simulink library "commdigpbnd"  (Simulink 5.0)
undefined symbols (not defined in the file or in its folder): j, Offset, T
libraries: commdigbbnd x13, commanapbnd x11, commutil x9, commdigpbnd x3, commsource x1
settings Model: Creator=tdelve  LastModifiedBy=mmclerno

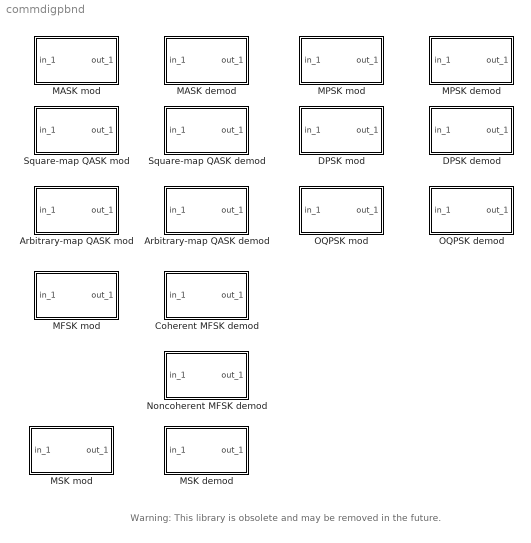
== system commdigpbnd ==
  note: Warning: This library is obsolete and may be removed in the future.
  Arbitrary-map QASK demod : Subsystem  mask(Passband A-map QASK demodulation){y1=real(exp(j*[0:8-1]/8*pi*2)), y2=imag(exp(j*[0:8-1]/8*pi*2)), td=0.1, Fc=100, Ph=0, ts=0.001}
      mask prompts: y1 "Vector of in-phase component:"; y2 "Vector of quadrature component:"; td "Symbol interval (sec):"; Fc "Carrier frequency (Hz):"; Ph "Initial phase (rad):"; ts "Sample time (sec):"
      mask help: Demodulate a QASK modulated signal with user-defined arbitrary constellation.
      mask init:
      | [num,den]=butter(5,Fc*2*ts);
      mask Help: This block demodulates a QASK modulated signal using user-defined arbitrary constellation. The arbitrary defined map is given in in-phase and quadrature component vector. The vector length of in-phase and quadrature components should have the same length. This block uses a default lowpass filter, which is [num,den]=butter(5,Fc*2*ts). Ungroup this block to define your own filter.
      mask Display:
      | plot(0,0,100,100,[5+1.5*[[0:.8:10] [10 20] [20:.8:30]] 50 50 50 50+15*[0 1 1 2 2 3]],[85+10*[sin([0:.8:10]*pi*2/5) 0 0 sin([20:.8:30]*pi*2/5)] 85 99 75 85+8*[1 1 -1 -1 1 1]]);
      | disp('\nPassband\nA-QASK')
  Arbitrary-map QASK mod : Subsystem  mask(Passband A-map QASK modulation){y1=real(exp(j*[0:8-1]/8*pi*2)), y2=imag(exp(j*[0:8-1]/8*pi*2)), td=0.1, Fc=100, Ph=0, ts=0.001}
      mask prompts: y1 "Vector of in-phase component:"; y2 "Vector of quadrature component:"; td "Symbol interval (sec):"; Fc "Carrier frequency (Hz):"; Ph "Initial phase (rad):"; ts "Sample time (sec):"
      mask help: Modulate the input digital signal using quadrature amplitude shift keying method with arbitrary constellation.
      mask Help: This block modulates a digital signal using QASK method with user-defined arbitrary constellation. The vector length of the in-phase and quadrature components vector should have the same length. The inputs are integers in the range [0, M-1], where M is the M-ary number. When the symbol interval is a two-element vector, the second element is the offset (default 0).
      mask Display:
      | plot(0,0,100,100,[5+15*[0 1 1 2 2 3] 50 50 50 50+1.5*[[0:.8:10] [10 20] [20:.8:30]]],[85+8*[1 1 -1 -1 1 1] 85 99 75 85+10*[sin([0:.8:10]*pi*2/5) 0 0 sin([20:.8:30]*pi*2/5)]]);
      | disp('\nPassband\nA-QASK')
  Coherent MFSK demod : Subsystem  mask(Passband MFSK demodulation){M=8, Ton=8/.1/5, td=0.1, Fc=100, Ph=0, ts=0.001}
      mask prompts: M "M-ary number (output digits in range [0, M-1]):"; Ton "Tone space (Hz):"; td "Symbol interval (sec):"; Fc "Carrier frequency (Hz):"; Ph "Initial phase (rad):"; ts "Sample time (sec):"
      mask help: Demodulate a MFSK modulated signal using coherent demodulation method.
      mask Help: This block demodulates a MFSK modulated signal using coherent method. The coherence demodulation method is phase sensitive. The tone space is the frequency distance between two consecutive digit after the modulation. The inputs are integers in the range [0, M-1], where M is the M-ary number. When the symbol interval is a two-element vector, the second element is the offset (default 0).
      mask Display:
      | plot(0,0,100,100,[5+1.5*[[0:.8:10] [10:1.6:20] [20:.8:30]] 50 50 50 50+15*[0 1 1 2 2 3]],[85+10*[sin([0:.8:10]*pi*2/5) sin([10:1.6:20]*pi/5) sin([20:.8:30]*pi*2/5)] 85 99 75 85+8*[1 1 -1 -1 1 1]]);
      | disp('\nPassband\nCohe MFSK')
  DPSK demod : Subsystem  mask(Passband DPSK demodulation){td=0.1, Fc=100, Ph=0, ts=0.001}
      mask prompts: td "Symbol interval (sec):"; Fc "Carrier frequency (Hz):"; Ph "Initial phase (rad):"; ts "Sample time (sec):"
      mask help: Demodulate a DPSK modulated signal.
      mask Help: This block demodulates a DPSK modulated signal using the digital MPSK Demod block and the Differential Decoder block. The input is a modulated analog signal and the output is a demodulated binary signal. Match the parameters to the ones used in the corresponding DPSK Mod block. The offset value in Symbol interval can be different.
      mask Display:
      | plot(0,0,100,100,[5+1.5*[[0:.8:10] [10:1.6:20] [20:.8:30]] 50 50 50 50+15*[0 1 1 2 2 3]],[85+10*[sin([0:.8:10]*pi*2/5) sin([10:1.6:20]*pi/5) sin([20:.8:30]*pi*2/5)] 85 99 75 85+8*[1 1 -1 -1 1 1]]);
      | disp('\nPassband\nDPSK')
  DPSK mod : Subsystem  mask(Passband DPSK modulation){td=0.1, Fc=100, Ph=0, ts=0.001}
      mask prompts: td "Symbol interval (sec):"; Fc "Carrier frequency (Hz):"; Ph "Initial phase (rad):"; ts "Sample time (sec):"
      mask help: Modulate the input signal using differential phase shift keying method.
      mask Help: This block modulates a digital signal with a given carrier frequency using the DPSK method. The input to this block is a binary signal. When the symbol interval is a two-element vector, the second element is the offset (default is 0). The output is a modulated analog signal with a maximum amplitude equal to 1.
      mask Display:
      | plot(0,0,100,100,[5+15*[0 1 1 2 2 3] 50 50 50 50+1.5*[[0:.8:10] [10:1.6:20] [20:.8:30]]],[85+8*[1 1 -1 -1 1 1] 85 99 75 85+10*[sin([0:.8:10]*pi*2/5) sin([10:1.6:20]*pi/5) sin([20:.8:30]*pi*2/5)]]);
      | disp('\nPassband\nDPSK')
  MASK demod : Subsystem  mask(Passband MASK demodulation){M=8, td=0.1, Fc=100, Ph=0, ts=0.001}
      mask prompts: M "M-ary number (output integer in range [0, M-1]):"; td "Symbol interval (sec):"; Fc "Carrier Frequency (Hz):"; Ph "Initial phase (rad):"; ts "Sample time (sec):"
      mask help: Demodulate a MASK modulated signal.
      mask init:
      | [num,den]=butter(5,Fc*2*ts);
      mask Help: This block demodulates a MASK modulated signal. The output signals are digits in range [0, M-1]. When the symbol interval is a two element vector, the second element is the offset (default 0). A default lowpass filter is used in the demodulation, which is [num, den]=butter(5, Fc*2*ts). Ungroup this block to specify the numerator and denominator of the lowpass filter.
      mask Display:
      | plot(0,0,100,100,[5+1.5*[[0:.8:10] [10 20] [20:.8:30]] 50 50 50 50+15*[0 1 1 2 2 3]],[85+10*[sin([0:.8:10]*pi*2/5) 0 0 sin([20:.8:30]*pi*2/5)] 85 99 75 85+8*[1 1 -1 -1 1 1]]);
      | disp('\nPassband\nMASK');
  MASK mod : Subsystem  mask(Passband MASK modulation){M=8, td=0.1, Fc=100, Ph=0, ts=0.001}
      mask prompts: M "M-ary number (input integer in range [0, M-1]):"; td "Input symbol interval (sec):"; Fc "Carrier frequency (Hz):"; Ph "Carrier initial phase (rad):"; ts "Sample time (sec):"
      mask help: Modulate the input digital signal using M-ary amplitude shift keying method.
      mask Help: This block modulates a digital signal using MASK method. The inputs are integers in the range [0, M-1], where M is the M-ary number. When the symbol interval is a two-element vector, the second element is the offset (default 0). The block keeps the input value at the offset time point for the entire interval.
      mask Display:
      | plot(0,0,100,100,[5+15*[0 1 1 2 2 3] 50 50 50 50+1.5*[[0:.8:10] [10 20] [20:.8:30]]],[85+8*[1 1 -1 -1 1 1] 85 99 75 85+10*[sin([0:.8:10]*pi*2/5) 0 0 sin([20:.8:30]*pi*2/5)]]);
      | disp('\nPassband\nMASK')
  MFSK mod : Subsystem  mask(Passband FSK modulation){Ton=8/.1/5, td=0.1, Fc=100, Ph=0, ts=0.001}
      mask prompts: Ton "Tone space(Hz):"; td "Symbol interval (sec):"; Fc "Carrier frequency (Hz):"; Ph "Initial phase (rad):"; ts "Sample time (sec):"
      mask help: Modulate the input digital signal using M-ary frequency shift keying method.
      mask Help: This block modulates a digital signal using FSK method. The modulation resets the modulation phase to be the specified initial phase at the beginning of each digit. Tone space is the frequency distance between two consecutive digits after modulation. The output signal has its frequency in the range [Fc, Fc + Tone_space*Max_In_Value], where Fc is the carrier frequency.
      mask Display:
      | plot(0,0,100,100,[5+15*[0 1 1 2 2 3] 50 50 50 50+1.5*[[0:.8:10] [10:1.6:20] [20:.8:30]]],[85+8*[1 1 -1 -1 1 1] 85 99 75 85+10*[sin([0:.8:10]*pi*2/5) sin([10:1.6:20]*pi/5) sin([20:.8:30]*pi*2/5)]]);
      | disp('\nPassband\nMFSK');
  MPSK demod : Subsystem  mask(Passband MPSK demodulation){M=8, td=0.1, Fc=100, Ph=0, ts=0.001}
      mask prompts: M "M-ary number (output integer in range [0, M-1]):"; td "Symbol interval (sec):"; Fc "Carrier frequency (Hz):"; Ph "Initial phase (rad):"; ts "Sample time (sec):"
      mask help: Demodulate a MPSK modulated signal using correlation method.
      mask Help: This block demodulates a MPSK modulated signal using correlation method. The output signals are digits in range [0, M-1], where M is the M-ary number. When the symbol interval is a two-element vector, the second element is the offset (default 0).
      mask Display:
      | plot(0,0,100,100,[5+1.5*[[0:.8:10] [10:1.6:20] [20:.8:30]] 50 50 50 50+15*[0 1 1 2 2 3]],[85+10*[sin([0:.8:10]*pi*2/5) sin([10:1.6:20]*pi/5) sin([20:.8:30]*pi*2/5)] 85 99 75 85+8*[1 1 -1 -1 1 1]]);
      | disp('\nPassband\nMPSK')
  MPSK mod : Subsystem  mask(Passband MPSK modulation){M=8, td=0.1, Fc=100, Ph=0, ts=0.001}
      mask prompts: M "M-ary number (input integer in range [0, M-1]):"; td "Symbol interval (sec):"; Fc "Carrier frequency (Hz):"; Ph "Initial phase (rad):"; ts "Sample time (sec):"
      mask help: Modulate the input signal using M-ary phase shift keying method.
      mask Help: This block modulates a digital signal with a given carrier frequency using MPSK method. The inputs are integers in the range [0, M-1], where M is the M-ary number. When the symbol interval is a two element vector, the second element is the offset (default 0). The block keeps the input value at the offset time point for the entire interval.
      mask Display:
      | plot(0,0,100,100,[5+15*[0 1 1 2 2 3] 50 50 50 50+1.5*[[0:.8:10] [10:1.6:20] [20:.8:30]]],[85+8*[1 1 -1 -1 1 1] 85 99 75 85+10*[sin([0:.8:10]*pi*2/5) sin([10:1.6:20]*pi/5) sin([20:.8:30]*pi*2/5)]]);
      | disp('\nPassband\nMPSK')
  MSK demod : Subsystem  mask(Passband MSK demodulation){td=0.1, Fc=100, Ph=0, ts=0.001}
      mask prompts: td "Symbol interval (sec):"; Fc "Carrier frequency (Hz):"; Ph "Initial phase (rad):"; ts "Sample time (sec):"
      mask help: Demodulate an MSK modulated signal.
      mask init:
      | T(1)=td(1);T2=2*T(1);if length(td)>1,T(2)=td(2); else, T(2)=0;end
      mask Help: This block demodulates an MSK modulated signal. It uses a matched filter to process the input signal and detect the in-phase and quadrature components of the signal. The filtered output is fed to an OQPSK Demap block resulting in a binary signal. Match the parameters to the ones used in the corresponding MSK Mod block. The offset value in Symbol interval can be different.
      mask Display:
      | plot(0,0,100,100,[5+1.5*[[0:.8:10] [10 20] [20:.8:30]] 50 50 50 50+15*[0 1 1 2 2 3]],[85+10*[sin([0:.8:10]*pi*2/5) 0 0 sin([20:.8:30]*pi*2/5)] 85 99 75 85+8*[1 1 -1 -1 1 1]]);
      | disp('\nPassband\nMSK')
  MSK mod : Subsystem  mask(Passband MSK modulation){td=0.1, Fc=100, Ph=0, ts=0.001}
      mask prompts: td "Symbol interval (sec):"; Fc "Carrier frequency (Hz):"; Ph "Initial phase (rad):"; ts "Sample time (sec):"
      mask help: Modulate the input signal using minimum phase shift keying method.
      mask Help: This block modulates a digital signal with a given carrier frequency using the MSK method. It uses the OQPSK Map block to map the binary input signal to the in-phase and quadrature components. When the symbol interval is a two-element vector, the second element is the offset (default is 0). The output is a modulated analog signal with a maximum amplitude equal to 1.
      mask Display:
      | plot(0,0,100,100,[5+15*[0 1 1 2 2 3] 50 50 50 50+1.5*[[0:.8:10] [10:1.6:20] [20:.8:30]]],[85+8*[1 1 -1 -1 1 1] 85 99 75 85+10*[sin([0:.8:10]*pi*2/5) sin([10:1.6:20]*pi/5) sin([20:.8:30]*pi*2/5)]]);
      | disp('\nPassband\nMSK')
  Noncoherent MFSK demod : Subsystem  mask(Passband MPSK demodulation){M=8, Ton=8/.1/5, td=0.1, Fc=100, Ph=pi/6, ts=0.001}
      mask prompts: M "M-ary number (output digits in range [0, M-1]):"; Ton "Tone space (Hz):"; td "Symbol interval (sec):"; Fc "Carrier frequency (Hz):"; Ph "Initial phase (rad):"; ts "Sample time (sec):"
      mask help: Demodulate a MFSK modulated signal using noncoherent method.
      mask Help: This block demodulates a MFSK modulated signal using noncoherent method. The tone space is the frequency distance between two consecutive after the modulation. The inputs are integers in the range [0, M-1], where M is the M-ary number. When the symbol interval is a two-element vector, the second element is the offset (default 0).
      mask Display:
      | plot(0,0,100,100,[5+1.5*[[0:.8:10] [10:1.6:20] [20:.8:30]] 50 50 50 50+15*[0 1 1 2 2 3]],[85+10*[sin([0:.8:10]*pi*2/5) sin([10:1.6:20]*pi/5) sin([20:.8:30]*pi*2/5)] 85 99 75 85+8*[1 1 -1 -1 1 1]]);
      | disp('\nPassband\nNonc MFSK')
  OQPSK demod : Subsystem  mask(Passband OQPSK demodulation){td=0.1, Fc=100, Ph=0, ts=0.001}
      mask prompts: td "Symbol interval (sec):"; Fc "Carrier frequency (Hz):"; Ph "Initial phase (rad):"; ts "Sample time (sec):"
      mask help: Demodulate an OQPSK modulated signal.
      mask init:
      | [num,den]=butter(5,Fc*2*ts);NIR=4;AIR=1/sqrt(2);PIR=pi/4;
      mask Help: This block demodulates an OQPSK modulated signal. The inputs are the in-phase and quadrature components of the QAM demodulated (QADM) signal. The output is a scalar binary signal with sample time T.
      mask Display:
      | plot(0,0,100,100,[5+1.5*[[0:.8:10] [10 20] [20:.8:30]] 50 50 50 50+15*[0 1 1 2 2 3]],[85+10*[sin([0:.8:10]*pi*2/5) 0 0 sin([20:.8:30]*pi*2/5)] 85 99 75 85+8*[1 1 -1 -1 1 1]]);
      | disp('\nPassband\nOQPSK')
  OQPSK mod : Subsystem  mask(Passband OQPSK modulation){td=0.1, Fc=100, Ph=0, ts=0.001}
      mask prompts: td "Symbol interval (sec):"; Fc "Carrier frequency (Hz):"; Ph "Initial phase (rad):"; ts "Sample time (sec):"
      mask help: Modulate the input signal using offset quadrature phase shift keying method.
      mask Help: This block modulates a digital signal with a given carrier frequency using the OQPSK method. The input to this block is a binary signal. When the symbol interval is a two-element vector, the second element is the offset (default is 0). The block uses the OQPSK Map block before feeding the signal to the QAM block. The output is a modulated analog signal with maximum amplitude equal to 1.
      mask Display:
      | plot(0,0,100,100,[5+15*[0 1 1 2 2 3] 50 50 50 50+1.5*[[0:.8:10] [10:1.6:20] [20:.8:30]]],[85+8*[1 1 -1 -1 1 1] 85 99 75 85+10*[sin([0:.8:10]*pi*2/5) sin([10:1.6:20]*pi/5) sin([20:.8:30]*pi*2/5)]]);
      | disp('\nPassband\nOQPSK')
  Square-map QASK demod : Subsystem  mask(Passband S-QASK demodulation){M=8, td=0.1, Fc=100, Ph=0, ts=0.001}
      mask prompts: M "M-ary number (output integer in range [0 M-1]):"; td "Symbol interval (sec):"; Fc "Carrier Frequency (Hz):"; Ph "Initial phase (rad):"; ts "Sample time (sec):"
      mask help: Demodulate a QASK modulated signal using square constellation.
      mask init:
      | [num,den]=butter(5,Fc*2*ts);
      mask Help: This block demodulates a MQASK modulated signal. The output signals are digits in the range [0, M-1]. When the symbol interval is a two-element vector, the second element is the offset (default 0). A default lowpass filter is used in the demodulation, which is [num, den]=butter(5, Fc*2*ts). Ungroup this block to specify the numerator and denominator of the lowpass filter.
      mask Display:
      | plot(0,0,100,100,[5+1.5*[[0:.8:10] [10 20] [20:.8:30]] 50 50 50 50+15*[0 1 1 2 2 3]],[85+10*[sin([0:.8:10]*pi*2/5) 0 0 sin([20:.8:30]*pi*2/5)] 85 99 75 85+8*[1 1 -1 -1 1 1]]);
      | disp('\nPassband\nS-QASK')
  Square-map QASK mod : Subsystem  mask(Passband S-QASK modulation){M=8, td=0.1, Fc=100, Ph=0, ts=0.001}
      mask prompts: M "M-ary number (input digits in range [0, M-1]):"; td "Symbol interval (sec):"; Fc "Carrier frequency (Hz):"; Ph "Initial phase (rad):"; ts "Sample time (sec):"
      mask help: Modulate the input signal using quadrature amplitude shift keying modulation method with square constellation.
      mask Help: This block modulates a digital signal using QASK method with square constellation. The inputs are integers in the range [0, M-1], where M is the M-ary number, which is M=2^K. K is an integer. When the symbol interval is a two element vector, the second element is the offset (default 0).
      mask Display:
      | plot(0,0,100,100,[5+15*[0 1 1 2 2 3] 50 50 50 50+1.5*[[0:.8:10] [10 20] [20:.8:30]]],[85+8*[1 1 -1 -1 1 1] 85 99 75 85+10*[sin([0:.8:10]*pi*2/5) 0 0 sin([20:.8:30]*pi*2/5)]]);
      | disp('\nPassband\nS-QASK')

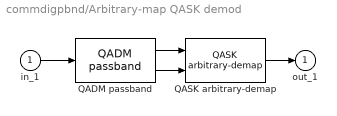
== system commdigpbnd/Arbitrary-map QASK demod ==
  in_1 : Inport
  QADM passband : commanapbnd/QADM passband  Fc=Fc  num=num  den=den  Ph=Ph  ts=ts
  QASK arbitrary-demap : commdigbbnd/A-map QASK demod baseband/QASK arbitrary-demap  y1=y1  y2=y2  td=td
  out_1 : Outport  InitialOutput=0
  wires:
  QADM passband/2 -> QASK arbitrary-demap/2
  QADM passband/1 -> QASK arbitrary-demap/1
  QASK arbitrary-demap/1 -> out_1/1
  in_1/1 -> QADM passband/1

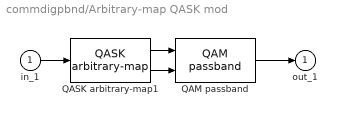
== system commdigpbnd/Arbitrary-map QASK mod ==
  in_1 : Inport
  QAM passband : commanapbnd/QAM passband  Fc=Fc  Ph=Ph  ts=ts
  QASK arbitrary-map1 : commdigbbnd/A-map QASK mod baseband/QASK arbitrary-map  y1=y1  y2=y2  td=td
  out_1 : Outport  InitialOutput=0
  wires:
  in_1/1 -> QASK arbitrary-map1/1
  QAM passband/1 -> out_1/1
  QASK arbitrary-map1/1 -> QAM passband/1
  QASK arbitrary-map1/2 -> QAM passband/2

== system commdigpbnd/Coherent MFSK demod ==
  in_1 : Inport
  Coh MFSK demod corr passband : Subsystem  mask(Passband coherent MFSK correlation){N=M, Ton=Ton, td=td, Ph=Ph, ts=ts}
      mask prompts: N "M-ary number (input in range [0, M-1]):"; Ton "Tone space (Hz):"; td "Symbol interval and offset (sec):"; Ph "Carrier frequency (Hz):"; ts "Initial phase (rad):"
      mask help: Compute MFSK correlation. Take MFSK modulated signal. Output a vector of correlation result.
      mask init:
      | pi2=2*pi;Fc=@4*pi2;sft=[0:N-1]*Ton*pi2;
      mask Help: This block calculates the coherent correlation value of the input signal with a vector of sinusoidal signals. These sinusoidal signals have their frequency the same as that of FM modulated signal of possible resulting digits. The output is an M length vector. M is the M-ary number. The MFSK demodulation result is the index of the largest output, using the Min/max demap block. The computation is phase sensitive.
      mask Display: disp('Coh corr\nMFSK dm')
  Min/max index : commdigbbnd/Coh MFSK demod baseband/Min//max index  td=td  mima='max'
  out_1 : Outport  InitialOutput=0
  wires:
  Min/max index/1 -> out_1/1
  in_1/1 -> Coh MFSK demod corr passband/1(in_1)
  Coh MFSK demod corr passband/1(out_1) -> Min/max index/1

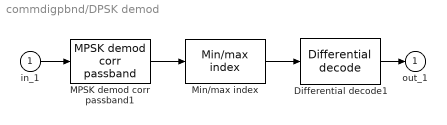
== system commdigpbnd/DPSK demod ==
  in_1 : Inport
  Differential decode1 : commutil/Differential decode  td=td
  MPSK demod corr passband1 : commdigpbnd/MPSK demod/MPSK demod corr passband  N=2  td=td  Ph=Ph  ts=ts  MaskParam3=Fc
  Min/max index : commdigbbnd/Coh MFSK demod baseband/Min//max index  td=td  mima='max'
  out_1 : Outport  InitialOutput=0
  wires:
  in_1/1 -> MPSK demod corr passband1/1
  MPSK demod corr passband1/1 -> Min/max index/1
  Min/max index/1 -> Differential decode1/1
  Differential decode1/1 -> out_1/1

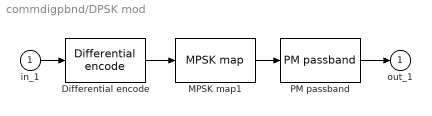
== system commdigpbnd/DPSK mod ==
  in_1 : Inport
  Differential encode : commutil/Differential encode  td=td
  MPSK map1 : commdigbbnd/MPSK mod baseband/MPSK map  td=td  MaskParam1=2
  PM passband : commanapbnd/PM passband  Fc=Fc  Ph=Ph  Kc=1  td=td
  out_1 : Outport  InitialOutput=0
  wires:
  MPSK map1/1 -> PM passband/1
  PM passband/1 -> out_1/1
  in_1/1 -> Differential encode/1
  Differential encode/1 -> MPSK map1/1

== system commdigpbnd/MASK demod ==
  in_1 : Inport
  DSB-SC-ADM passband : commanapbnd/DSB-SC-ADM passband  MaskParam1=Fc  MaskParam2=num  MaskParam3=den  MaskParam4=Ph  MaskParam5=ts
  MASK demap1 : commdigbbnd/MASK demod baseband/MASK demap  M=M  td=td
  out_1 : Outport  InitialOutput=0
  wires:
  MASK demap1/1 -> out_1/1
  DSB-SC-ADM passband/1 -> MASK demap1/1
  in_1/1 -> DSB-SC-ADM passband/1

== system commdigpbnd/MASK mod ==
  in_1 : Inport
  DSB-SC AM passband : commanapbnd/DSB-SC AM passband  MaskParam1=Fc  MaskParam2=Ph  MaskParam3=ts
  MASK map : commdigbbnd/MASK mod baseband/MASK map  N=M  td=td
  out_1 : Outport  InitialOutput=0
  wires:
  DSB-SC AM passband/1 -> out_1/1
  in_1/1 -> MASK map/1
  MASK map/1 -> DSB-SC AM passband/1

== system commdigpbnd/MFSK mod ==
  in_1 : Inport
  FM passband : commanapbnd/FM passband  Fc=Fc  Ph=Ph  HzPerV=1  ts=ts  td=td
  MFSK map : commdigbbnd/MFSK mod baseband/MFSK map  Ton=Ton  td=td
  out_1 : Outport  InitialOutput=0
  wires:
  in_1/1 -> MFSK map/1
  FM passband/1 -> out_1/1
  MFSK map/1 -> FM passband/1

== system commdigpbnd/MPSK demod ==
  in_1 : Inport
  MPSK demod corr passband : Subsystem  mask(Passband MPSK coherent MPSK correlation){N=M, td=td, Ph=Ph, ts=ts}
      mask prompts: N "M-ary number (integer in range [0, M-1]):"; td "Symbol interval and offset (sec):"; Ph "Carrier frequency (Hz):"; ts "Initial phase (rad):"
      mask help: Compute MPSK correlation. Take MPSK modulated signal. Output a vector of correlation result.
      mask init:
      | pi2=2*pi;sft=[0:N-1]*pi2/N;Fc=@3*pi2;
      mask Help: This block calculates the correlation value of the input signal with a vector of sinusoidal signals. These sinusoidal signals have their phase shift the same as that of PM modulated signal of possible resulting digits. The output is an M length vector. M is the M-ary number. The MPSK demodulation result is the index of the largest output, using the Min/max demap block. The computation is phase sensitive.
      mask Display: disp('Corr MPSK\ndemod')
  Min/max index : commdigbbnd/Coh MFSK demod baseband/Min//max index  td=td  mima='max'
  out_1 : Outport  InitialOutput=0
  wires:
  Min/max index/1 -> out_1/1
  in_1/1 -> MPSK demod corr passband/1(in_1)
  MPSK demod corr passband/1(out_1) -> Min/max index/1

== system commdigpbnd/MPSK mod ==
  in_1 : Inport
  MPSK map : commdigbbnd/MPSK mod baseband/MPSK map  td=td  MaskParam1=M
  PM passband : commanapbnd/PM passband  Fc=Fc  Ph=Ph  Kc=1  td=td
  out_1 : Outport  InitialOutput=0
  wires:
  in_1/1 -> MPSK map/1
  PM passband/1 -> out_1/1
  MPSK map/1 -> PM passband/1

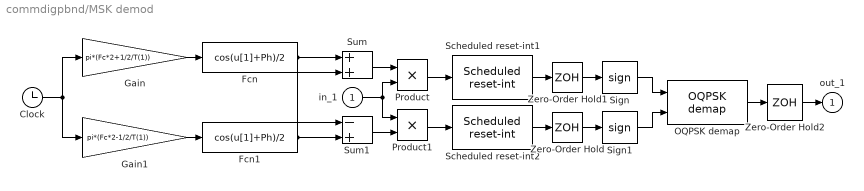
== system commdigpbnd/MSK demod ==
  in_1 : Inport
  Clock : Clock
      settings: Decimation=10
  Fcn : Fcn  Expr=cos(u[1]+Ph)/2
  Fcn1 : Fcn  Expr=cos(u[1]+Ph)/2
  Gain : Gain  Gain=pi*(Fc*2+1/2/T(1))  SaturateOnIntegerOverflow=on
  Gain1 : Gain  Gain=pi*(Fc*2-1/2/T(1))  SaturateOnIntegerOverflow=on
  OQPSK demap : commdigpbnd/OQPSK demod/OQPSK demap  td=td
  Product : Product  SaturateOnIntegerOverflow=on  InputSameDT=on
  Product1 : Product  SaturateOnIntegerOverflow=on  InputSameDT=on
  Scheduled reset-int1 : commutil/Scheduled reset-int  td=[2*T(1), T(1)+T(2)]  ts=ts  limit=Inf
  Scheduled reset-int2 : commutil/Scheduled reset-int  td=[2*T(1), T(2)]  ts=ts  limit=Inf
  Sign : Signum
  Sign1 : Signum
  Sum : Sum  SaturateOnIntegerOverflow=on  InputSameDT=on
  Sum1 : Sum  Inputs=-+  SaturateOnIntegerOverflow=on  InputSameDT=on
  Zero-Order Hold : ZeroOrderHold  SampleTime=[2*T(1), T(2)]
  Zero-Order Hold1 : ZeroOrderHold  SampleTime=[2*T(1), T(1)+T(2)]
  Zero-Order Hold2 : ZeroOrderHold  SampleTime=T
  out_1 : Outport  InitialOutput=0
  wires:
  Sign1/1 -> OQPSK demap/2
  Sign/1 -> OQPSK demap/1
  Zero-Order Hold/1 -> Sign1/1
  Zero-Order Hold1/1 -> Sign/1
  Scheduled reset-int2/1 -> Zero-Order Hold/1
  Scheduled reset-int1/1 -> Zero-Order Hold1/1
  Product1/1 -> Scheduled reset-int2/1
  Product/1 -> Scheduled reset-int1/1
  in_1/1 -> Product1/1, Product/2
  Fcn/1 -> Sum1/1, Sum/1
  Gain/1 -> Fcn/1
  Fcn1/1 -> Sum1/2, Sum/2
  Gain1/1 -> Fcn1/1
  Sum/1 -> Product/1
  Sum1/1 -> Product1/2
  Clock/1 -> Gain1/1, Gain/1
  OQPSK demap/1 -> Zero-Order Hold2/1
  Zero-Order Hold2/1 -> out_1/1

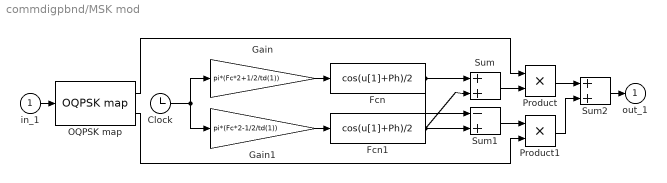
== system commdigpbnd/MSK mod ==
  in_1 : Inport
  Clock : Clock
      settings: Decimation=10
  Fcn : Fcn  Expr=cos(u[1]+Ph)/2
  Fcn1 : Fcn  Expr=cos(u[1]+Ph)/2
  Gain : Gain  Gain=pi*(Fc*2+1/2/td(1))  SaturateOnIntegerOverflow=on
  Gain1 : Gain  Gain=pi*(Fc*2-1/2/td(1))  SaturateOnIntegerOverflow=on
  OQPSK map : commdigpbnd/OQPSK mod/OQPSK map  T=td
  Product : Product  SaturateOnIntegerOverflow=on  InputSameDT=on
  Product1 : Product  SaturateOnIntegerOverflow=on  InputSameDT=on
  Sum : Sum  SaturateOnIntegerOverflow=on  InputSameDT=on
  Sum1 : Sum  Inputs=-+  SaturateOnIntegerOverflow=on  InputSameDT=on
  Sum2 : Sum  SaturateOnIntegerOverflow=on  InputSameDT=on
  out_1 : Outport  InitialOutput=0
  wires:
  in_1/1 -> OQPSK map/1
  Gain/1 -> Fcn/1
  Clock/1 -> Gain1/1, Gain/1
  Fcn/1 -> Sum1/1, Sum/1
  Gain1/1 -> Fcn1/1
  Fcn1/1 -> Sum1/2, Sum/2
  Sum1/1 -> Product1/1
  Sum/1 -> Product/2
  Product/1 -> Sum2/1
  Product1/1 -> Sum2/2
  OQPSK map/2 -> Product1/2
  OQPSK map/1 -> Product/1
  Sum2/1 -> out_1/1

== system commdigpbnd/Noncoherent MFSK demod ==
  in_1 : Inport
  Min/max index : commdigbbnd/Coh MFSK demod baseband/Min//max index  td=td  mima='max'
  Non-coh MFSK dm corr passband : Subsystem  mask(Passband non-coherent MFSK correlation){N=M, Ton=Ton, td=td, Ph=Ph, ts=ts}
      mask prompts: N "M-ary number (input in range [0, M-1]):"; Ton "Tone space (Hz):"; td "Symbol interval and offset (sec):"; Ph "Carrier frequency (Hz):"; ts "Initial phase (rad):"
      mask help: Compute MFSK correlation. Take MFSK modulated signal. Output a vector of correlation result.
      mask init:
      | pi2=2*pi;Fc=@4*pi2;sft=[0:N-1]*Ton*pi2;
      mask Help: This block calculates the noncoherent correlation value of the input signal with a vector of sinusoidal signals. These sinusoidal signals have their frequency the same as that of FM modulated signal of possible resulting digits. The output is an M length vector. M is the M-ary number. The MFSK demodulation result is the index of the largest output, using the Min/max demap block.
      mask Display: disp('Noncoh corr\nMFSK dm')
  out_1 : Outport  InitialOutput=0
  wires:
  Min/max index/1 -> out_1/1
  in_1/1 -> Non-coh MFSK dm corr passband/1(in_1)
  Non-coh MFSK dm corr passband/1(out_1) -> Min/max index/1

== system commdigpbnd/OQPSK demod ==
  in_1 : Inport
  OQPSK demap : Subsystem  mask(OQPSK demap){td=td}
      mask prompts: td "Symbol interval and offset (sec):"
      mask help: Reverse the OQPSK map. Input in-phase and quadrature components from the two inputs and output the demapped signal.
      mask init:
      | N=4;A=1/sqrt(2);P=pi/4;y1=apkconst(N,A,P);y2=imag(y1);y1=real(y1);T=td(1);T2=2*T;if length(td)>1,Offset=td(2); else, Offset=0;end
      mask Help: This block demaps an OQPSK mapped signal. You can place this block after a QAM demodulation (QADM) block. The two inputs are the in-phase and quadrature elements of the QAM demodulated  (QADM)signal. The output is a binary signal with sample time T.
      mask Display: disp('OQPSK\ndemap')
  QADM passband : commanapbnd/QADM passband  Fc=Fc  num=num  den=den  Ph=Ph  ts=ts
  out_1 : Outport  InitialOutput=0
  wires:
  in_1/1 -> QADM passband/1
  QADM passband/1 -> OQPSK demap/1(real)
  QADM passband/2 -> OQPSK demap/2(imag)
  OQPSK demap/1(out_1) -> out_1/1

== system commdigpbnd/OQPSK mod ==
  in_1 : Inport
  OQPSK map : Subsystem  mask(OQPSK map){T=td}
      mask prompts: T "Symbol interval (sec):"
      mask help: The input binary signal, with sample time T, is mapped into the 1/-1 value in-phase component with sample time 2T and offset 0, and into the quadrature component with sample time 2T and offset T.
      mask init:
      | if length(T)<2, T=[T, 0]; end;
      mask Help: This block maps the scalar binary input signal to the offset QPSK encoded signal. The value of the output of this block is either 1 or -1. The first output is the in-phase component. The second output of this block is the quadrature component. Note the difference between QPSK and OQPSK. This block does not introduce any delay.
      mask Display: disp('OQPSK\nmap')
  QAM passband : commanapbnd/QAM passband  Fc=Fc  Ph=Ph  ts=ts
  out_1 : Outport  InitialOutput=0
  wires:
  in_1/1 -> OQPSK map/1(In1)
  QAM passband/1 -> out_1/1
  OQPSK map/2(Out2) -> QAM passband/2
  OQPSK map/1(Out1) -> QAM passband/1

== system commdigpbnd/Square-map QASK demod ==
  in_1 : Inport
  QADM passband : commanapbnd/QADM passband  Fc=Fc  num=num  den=den  Ph=Ph  ts=ts
  QASK square-demap : commdigbbnd/S-map QASK demod baseband/QASK square-demap  N=M  td=td
  out_1 : Outport  InitialOutput=0
  wires:
  in_1/1 -> QADM passband/1
  QASK square-demap/1 -> out_1/1
  QADM passband/1 -> QASK square-demap/1
  QADM passband/2 -> QASK square-demap/2

== system commdigpbnd/Square-map QASK mod ==
  in_1 : Inport
  QAM passband : commanapbnd/QAM passband  Fc=Fc  Ph=Ph  ts=ts
  QASK square-map1 : commdigbbnd/S-map QASK mod baseband/QASK square-map  N=M  td=td
  out_1 : Outport  InitialOutput=0
  wires:
  in_1/1 -> QASK square-map1/1
  QAM passband/1 -> out_1/1
  QASK square-map1/2 -> QAM passband/2
  QASK square-map1/1 -> QAM passband/1

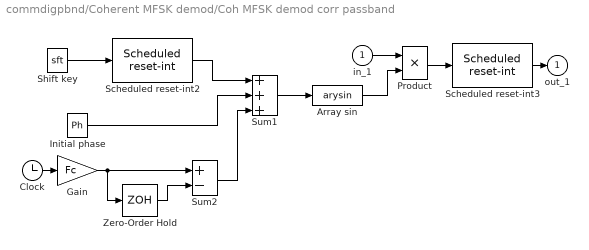
== system commdigpbnd/Coherent MFSK demod/Coh MFSK demod corr passband ==
  in_1 : Inport
  Array sin : S-Function  FunctionName=arysin  Parameters='cos'
  Clock : Clock
      settings: Decimation=10
  Gain : Gain  Gain=Fc  SaturateOnIntegerOverflow=on
  Initial phase : Constant  Value=Ph
  Product : Product  SaturateOnIntegerOverflow=on  InputSameDT=on
  Scheduled reset-int2 : commutil/Scheduled reset-int  td=td  ts=ts  limit=Inf
  Scheduled reset-int3 : commutil/Scheduled reset-int  td=td  ts=ts  limit=Inf
  Shift key : Constant  Value=sft
  Sum1 : Sum  Inputs=+++  SaturateOnIntegerOverflow=on  InputSameDT=on
  Sum2 : Sum  Inputs=+-  SaturateOnIntegerOverflow=on  InputSameDT=on
  Zero-Order Hold : ZeroOrderHold  SampleTime=td
  out_1 : Outport  InitialOutput=0
  wires:
  Scheduled reset-int3/1 -> out_1/1
  in_1/1 -> Product/1
  Product/1 -> Scheduled reset-int3/1
  Sum1/1 -> Array sin/1
  Array sin/1 -> Product/2
  Shift key/1 -> Scheduled reset-int2/1
  Scheduled reset-int2/1 -> Sum1/1
  Initial phase/1 -> Sum1/2
  Clock/1 -> Gain/1
  Sum2/1 -> Sum1/3
  Gain/1 -> Sum2/1, Zero-Order Hold/1
  Zero-Order Hold/1 -> Sum2/2

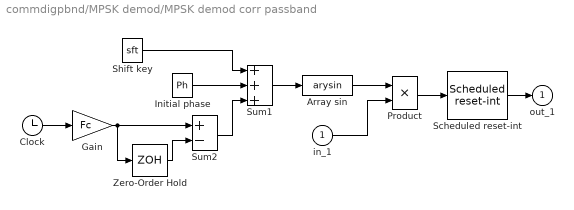
== system commdigpbnd/MPSK demod/MPSK demod corr passband ==
  in_1 : Inport
  Array sin : S-Function  FunctionName=arysin  Parameters='cos'
  Clock : Clock
      settings: Decimation=10
  Gain : Gain  Gain=Fc  SaturateOnIntegerOverflow=on
  Initial phase : Constant  Value=Ph
  Product : Product  SaturateOnIntegerOverflow=on  InputSameDT=on
  Scheduled reset-int : commutil/Scheduled reset-int  td=td  ts=ts  limit=Inf
  Shift key : Constant  Value=sft
  Sum1 : Sum  Inputs=+++  SaturateOnIntegerOverflow=on  InputSameDT=on
  Sum2 : Sum  Inputs=+-  SaturateOnIntegerOverflow=on  InputSameDT=on
  Zero-Order Hold : ZeroOrderHold  SampleTime=td
  out_1 : Outport  InitialOutput=0
  wires:
  in_1/1 -> Product/2
  Array sin/1 -> Product/1
  Zero-Order Hold/1 -> Sum2/2
  Gain/1 -> Zero-Order Hold/1, Sum2/1
  Sum2/1 -> Sum1/3
  Clock/1 -> Gain/1
  Initial phase/1 -> Sum1/2
  Shift key/1 -> Sum1/1
  Sum1/1 -> Array sin/1
  Product/1 -> Scheduled reset-int/1
  Scheduled reset-int/1 -> out_1/1

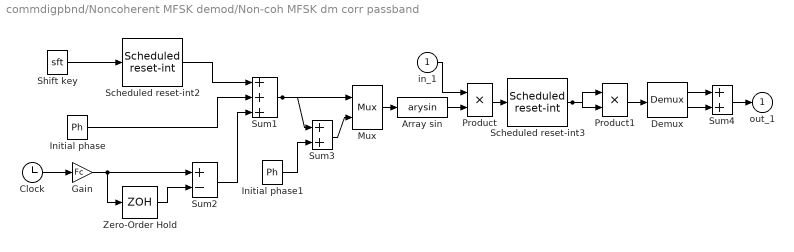
== system commdigpbnd/Noncoherent MFSK demod/Non-coh MFSK dm corr passband ==
  in_1 : Inport
  Array sin : S-Function  FunctionName=arysin  Parameters='cos'
  Clock : Clock
      settings: Decimation=10
  Demux : Demux  Outputs=[N N]
  Gain : Gain  Gain=Fc  SaturateOnIntegerOverflow=on
  Initial phase : Constant  Value=Ph
  Initial phase1 : Constant  Value=Ph
  Mux : Mux  Inputs=[N N]
  Product : Product  SaturateOnIntegerOverflow=on  InputSameDT=on
  Product1 : Product  SaturateOnIntegerOverflow=on  InputSameDT=on
  Scheduled reset-int2 : commutil/Scheduled reset-int  td=td  ts=ts  limit=Inf
  Scheduled reset-int3 : commutil/Scheduled reset-int  td=td  ts=ts  limit=Inf
  Shift key : Constant  Value=sft
  Sum1 : Sum  Inputs=+++  SaturateOnIntegerOverflow=on  InputSameDT=on
  Sum2 : Sum  Inputs=+-  SaturateOnIntegerOverflow=on  InputSameDT=on
  Sum3 : Sum  SaturateOnIntegerOverflow=on  InputSameDT=on
  Sum4 : Sum  SaturateOnIntegerOverflow=on  InputSameDT=on
  Zero-Order Hold : ZeroOrderHold  SampleTime=td
  out_1 : Outport  InitialOutput=0
  wires:
  Sum4/1 -> out_1/1
  in_1/1 -> Product/1
  Demux/2 -> Sum4/2
  Demux/1 -> Sum4/1
  Product1/1 -> Demux/1
  Scheduled reset-int3/1 -> Product1/2, Product1/1
  Product/1 -> Scheduled reset-int3/1
  Array sin/1 -> Product/2
  Mux/1 -> Array sin/1
  Sum3/1 -> Mux/2
  Initial phase1/1 -> Sum3/2
  Sum1/1 -> Mux/1, Sum3/1
  Zero-Order Hold/1 -> Sum2/2
  Gain/1 -> Sum2/1, Zero-Order Hold/1
  Sum2/1 -> Sum1/3
  Clock/1 -> Gain/1
  Initial phase/1 -> Sum1/2
  Scheduled reset-int2/1 -> Sum1/1
  Shift key/1 -> Scheduled reset-int2/1

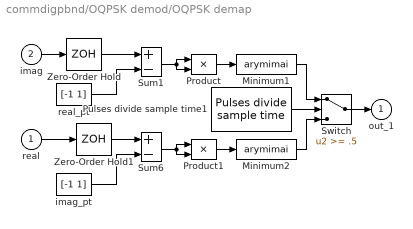
== system commdigpbnd/OQPSK demod/OQPSK demap ==
  real : Inport
  imag : Inport  Port=2
  Minimum1 : S-Function  FunctionName=arymimai  Parameters='min'
  Minimum2 : S-Function  FunctionName=arymimai  Parameters='min'
  Product : Product  SaturateOnIntegerOverflow=on  InputSameDT=on
  Product1 : Product  SaturateOnIntegerOverflow=on  InputSameDT=on
  Pulses divide sample time1 : commsource/Pulses divide sample time  samp_time=T2  out_divid=1  offset=Offset
  Sum1 : Sum  Inputs=+-  SaturateOnIntegerOverflow=on  InputSameDT=on
  Sum6 : Sum  Inputs=+-  SaturateOnIntegerOverflow=on  InputSameDT=on
  Switch : Switch  Threshold=.5  SaturateOnIntegerOverflow=on  InputSameDT=on
  Zero-Order Hold : ZeroOrderHold  SampleTime=[T2, Offset]
  Zero-Order Hold1 : ZeroOrderHold  SampleTime=[T2, Offset+T]
  imag_pt : Constant  Value=[-1 1]
  real_pt : Constant  Value=[-1 1]
  out_1 : Outport  InitialOutput=0
  wires:
  Pulses divide sample time1/1 -> Switch/2
  Zero-Order Hold/1 -> Sum1/1
  Zero-Order Hold1/1 -> Sum6/1
  imag_pt/1 -> Sum6/2
  Minimum2/1 -> Switch/3
  Minimum1/1 -> Switch/1
  Switch/1 -> out_1/1
  Product1/1 -> Minimum2/1
  Product/1 -> Minimum1/1
  Sum6/1 -> Product1/2, Product1/1
  Sum1/1 -> Product/2, Product/1
  real_pt/1 -> Sum1/2
  real/1 -> Zero-Order Hold1/1
  imag/1 -> Zero-Order Hold/1

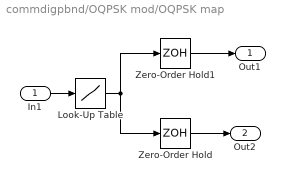
== system commdigpbnd/OQPSK mod/OQPSK map ==
  In1 : Inport
  Look-Up Table : Lookup  InputValues=[0 .5 .5 1]  OutputValues=[-1 -1 1 1]  SaturateOnIntegerOverflow=on
  Zero-Order Hold : ZeroOrderHold  SampleTime=[2*T(1), T(2)]
  Zero-Order Hold1 : ZeroOrderHold  SampleTime=[2*T(1), T(1)+T(2)]
  Out1 : Outport  InitialOutput=0
  Out2 : Outport  Port=2  InitialOutput=0
  wires:
  Look-Up Table/1 -> Zero-Order Hold1/1, Zero-Order Hold/1
  In1/1 -> Look-Up Table/1
  Zero-Order Hold1/1 -> Out1/1
  Zero-Order Hold/1 -> Out2/1
